simulink model "ModelMotS_dq_V2bis_FVC"  (R2018b)
settings: Solver=ode45  StartTime=0.0  StopTime=40  MaxStep=1e-4  RelTol=1e-4  EnableMultiTasking=on
values from neighbouring files (symbols this model uses):
  J = 0.045    [gen_sim_new_data_december.m]
  Lfr = 0.007    [gen_sim_new_data_december.m]
  Lfs = 0.007    [gen_sim_new_data_december.m]
  Lm = 0.153    [gen_sim_new_data_december.m]
  Lmt = 0.210    (= 0.21)    [gen_sim_new_data_december.m]
  Lr = 0.160    (= 0.16)    [gen_sim_new_data_december.m]
  Ls = 0.160    (= 0.16)    [gen_sim_new_data_december.m]
  np = 2    [gen_sim_new_data_december.m]
  P1 = 0.7    [gen_sim_new_data_december.m]
  P2 = 1.5    [gen_sim_new_data_december.m]
  Prinit = [ 0 ; 0 ]    [gen_sim_new_data_december.m]
  Psinit = [ 0 ; 0 ]    [gen_sim_new_data_december.m]
  Rr = 0.9    [gen_sim_new_data_december.m]
  Rs = 1.5    [gen_sim_new_data_december.m]
  thrinit = 0    [gen_sim_new_data_december.m]
  wL = 2*pi*0    (= 0)    [gen_sim_new_data_december.m]
  wrinit = 2*pi*0    (= 0)    [gen_sim_new_data_december.m]
undefined symbols (not defined in the file or in its folder): Data_Ts, DiscIntNeverNeededParam, Inom, Jm, Prdnom, SFC_Coeff, SLP_Coeff, Tpwm, Vnom, wCurr, wCurr_PI, wSpeed_PI, wSpeedEst, xiCurr_PI, xiSpeed_PI
libraries: simulink x5
(part 1 of 2)
settings Model: Creator=stbp106  LastModifiedBy=root
settings DataIOCC: LimitDataPoints=on  SaveFormat=Array
settings OptimizationCC: LifeSpan=inf
settings DebuggingCC: UnderspecifiedInitializationDetection=Classic  MergeDetectMultiDrivingBlocksExec=none  SolverPrmCheckMsg=warning  SFUnexpectedBacktrackingDiag=warning  SFNoUnconditionalDefaultTransitionDiag=warning  SFExecutionAtInitializationDiag=none
settings HardwareCC: ProdBitPerPointer=32  ProdBitPerSizeT=32  ProdBitPerPtrDiffT=32  ProdLargestAtomicFloat=None  ProdIntDivRoundTo=Undefined  ProdEndianess=Unspecified  ProdWordSize=32  ProdHWDeviceType=32-bit Generic
settings ModelReferenceCC: PropagateSignalLabelsOutOfModel=off
settings SFSimCC: SimUseLocalCustomCode=off
settings RTWCC: RTWUseLocalCustomCode=off
settings CodeAppCC: StateflowObjectComments=on
settings GRTTargetCC: TargetLangStandard=C89/C90 (ANSI)  GeneratePreprocessorConditionals=Disable all
settings ConfigComp: CovMetricSettings=dw  CovHtmlReporting=on  CovSaveCumulativeToWorkspaceVar=on  CovSaveSingleToWorkspaceVar=on  CovExternalEMLEnable=off  CovSFcnEnable=off

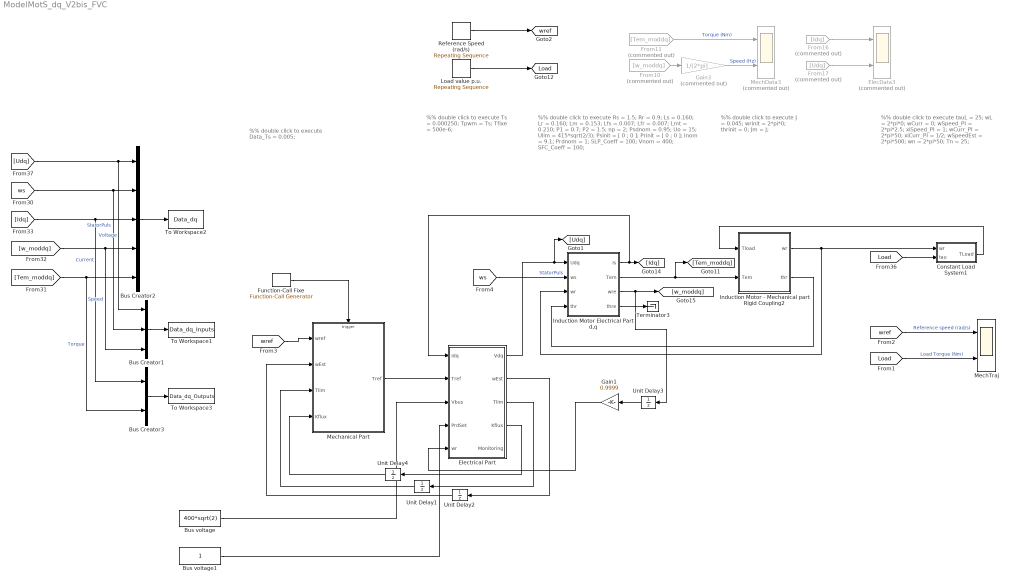
== system ModelMotS_dq_V2bis_FVC ==
  note: %% double click to execute
      |
      | Rs = 1.5; Rr = 0.9;
      | Ls = 0.160; Lr = 0.160; Lm = 0.153;
      | Lfs = 0.007; Lfr = 0.007; Lmt = 0.210; P1 = 0.7; P2 = 1.5;
      | np = 2;
      | Psdnom = 0.95; Uo = 15; Ulim = 415*sqrt(2/3);
      | Psinit = [ 0 ; 0 ]; Prinit = [ 0 ; 0 ];
      | Inom = 9.1; Prdnom = 1; SLP_Coeff = 100; Vnom = 400;
      | SFC_Coeff = 100;
  note: %% double click to execute
      |
      | J = 0.045;
      | wrinit = 2*pi*0;
      | thrinit = 0;
      | Jm = J;
  note: %% double click to execute
      |
      | tauL = 25;
      | wL = 2*pi*0;
      |
      | wCurr = 0;
      | wSpeed_PI = 2*pi*2.5; xiSpeed_PI = 1;
      | wCurr_PI = 2*pi*50; xiCurr_PI = 1/2;
      | wSpeedEst = 2*pi*500;
      |
      | wn = 2*pi*50;
      | Tn = 25;
  note: %% double click to execute
      |
      | Ts = 0.000250;
      | Tpwm = Ts;
      | Tfixe = 500e-6;
  note: %% double click to execute
      |
      | Data_Ts = 0.005;
  Bus Creator1 : BusCreator  Inputs=3
  Bus Creator2 : BusCreator  Inputs=5
  Bus Creator3 : BusCreator  Inputs=2
  Bus voltage : Constant  Value=400*sqrt(2)
  Bus voltage1 : Constant
  Constant Load System1 : Subsystem  Description=""
  ElecData3 : Scope  Commented=on  NumInputPorts=2
  Electrical Part : Subsystem
  From10 : From  Commented=on  GotoTag=w_moddq
  From11 : From  Commented=on  GotoTag=Tem_moddq
  From16 : From  Commented=on  GotoTag=Idq
  From17 : From  Commented=on  GotoTag=Udq
  Function-Call Fixe : simulink/Ports & Subsystems/Function-Call Generator  sample_time=Tfixe  numberOfIterations=1
  Gain1 : Gain  Gain=0.9999
  Gain3 : Gain  Commented=on  Gain=1/(2*pi)  SaturateOnIntegerOverflow=on  OutDataTypeStr=Inherit: Same as input  ParamDataTypeStr=Inherit: Same as input
  Induction Motor Electrical Part d,q : Subsystem  Description=""
  Induction Motor - Mechanical part Rigid Coupling2 : Subsystem  Description=""
  Load value p.u. : simulink/Sources/Repeating Sequence  rep_seq_t="[0        0.005         0.01        0.015         0.02        0.025         0.03        0.035         0.04        0.045         0.05        0.055         0.06        0.065         0.07        0.075         0.08        0.085         0.09        0.095          0.1        0.105         0.11        0.115         0.12        0.125         0.13        0.135         0.14        0.145         0.15        0.155         0.16        0.165         0.17        0.175         0.18        0.185         0.19        0.195          0.2        0.205         0.21        0.215         0.22        0.225         0.23        0.235         0.24        0.245         0.25        0.255         0.26        0.265         0.27        0.275         0.28        0.285         0.29        0.295          0.3        0.305         0.31        0.315         0.32        0.325         0.33        0.335         0.34        0.345         0.35        0.355         0.36        0.365         0.37        0.375         0.38        0.385         0.39        0.395          0.4        0.405         0.41        0.415         0.42        0.425         0.43        0.435         0.44        0.445         0.45        0.455         0.46        0.465         0.47        0.475         0.48        0.485         0.49        0.495          0.5        0.505         0.51        0.515         0.52        0.525         0.53        0.535         0.54        0.545         0.55        0.555         0.56        0.565         0.57        0.575         0.58        0.585         0.59        0.595          0.6        0.605         0.61        0.615         0.62        0.625         0.63        0.635         0.64        0.645         0.65        0.655         0.66        0.665         0.67        0.675         0.68        0.685         0.69        0.695          0.7        0.705         0.71        0.715         0.72        0.725         0.73        0.735         0.74        0.745         0.75        0.755         0.76        0.765         0.77        0.775         0.78        0.785         0.79        0.795          0.8        0.805         0.81        0.815         0.82        0.825         0.83        0.835         0.84        0.845         0.85        0.855         0.86        0.865         0.87        0.875         0.88        0.885         0.89        0.895          0.9        0.905         0.91        0.915         0.92        0.925         0.93        0.935         0.94        0.945         0.95        0.955         0.96        0.965         0.97        0.975         0.98        0.985         0.99        0.995            1        1.005         1.01        1.015         1.02        1.025         1.03        1.035         1.04        1.045         1.05        1.055         1.06        1.065         1.07        1.075         1.08        1.085         1.09        1.095          1.1        1.105         1.11        1.115         1.12        1.125         1.13        1.135         1.14        1.145         1.15        1.155         1.16        1.165         1.17        1.175         1.18        1.185         1.19        1.195          1.2        1.205         1.21        1.215         1.22        1.225         1.23        1.235         1.24        1.245         1.25        1.255         1.26        1.265         1.27        1.275         1.28        1.285         1.29        1.295          1.3        1.305         1.31        1.315         1.32        1.325         1.33        1.335         1.34        1.345         1.35        1.355         1.36        1.365         1.37        1.375         1.38        1.385         1.39        1.395          1.4        1.405         1.41        1.415         1.42        1.425         1.43        1.435         1.44        1.445         1.45        1.455         1.46        1.465         1.47        1.475         1.48        1.485         1.49        1.495          1.5        1.505         1.51        1.515         1.52        1.525         1.53        1.535 ...(+99990 chars)]"  rep_seq_y="[0            0            0            0            0            0            0            0            0            0            0            0            0            0            0            0            0            0            0            0            0            0            0            0            0            0            0            0            0            0            0            0            0            0            0            0            0            0            0            0            0            0            0            0            0            0            0            0            0            0            0            0            0            0            0            0            0            0            0            0            0            0            0            0            0            0            0            0            0            0            0            0            0            0            0            0            0            0            0            0            0            0            0            0            0            0            0            0            0            0            0            0            0            0            0            0            0            0            0            0            0            0            0            0            0            0            0            0            0            0            0            0            0            0            0            0            0            0            0            0            0            0            0            0            0            0            0            0            0            0            0            0            0            0            0            0            0            0            0            0            0            0            0            0            0            0            0            0            0            0            0            0            0            0            0            0            0            0            0            0            0            0            0            0            0            0            0            0            0            0            0            0            0            0            0            0            0            0            0            0            0            0            0            0            0            0            0            0            0            0            0            0            0            0            0            0            0            0            0            0            0            0            0            0            0            0            0            0            0            0            0            0            0            0            0            0            0            0            0            0            0            0            0            0            0            0            0            0            0            0            0            0            0            0            0            0            0            0            0            0            0            0            0            0            0            0            0            0            0            0            0            0            0            0            0            0            0            0            0            0            0            0            0            0            0            0            0            0            0            0            0            0            0            0            0            0            0            0            0            0            0            0            0            0            0            0            0            0            0            0            0            0            0            0            0            0            0            0            0            0            0            0            0            0            0            0            0            0 ...(+99990 chars)]"
  MechData3 : Scope  Commented=on  NumInputPorts=2
  MechTraj : Scope  NumInputPorts=2
  Mechanical Part : Subsystem
  Reference Speed (rad/s) : simulink/Sources/Repeating Sequence  rep_seq_t="[0        0.005         0.01        0.015         0.02        0.025         0.03        0.035         0.04        0.045         0.05        0.055         0.06        0.065         0.07        0.075         0.08        0.085         0.09        0.095          0.1        0.105         0.11        0.115         0.12        0.125         0.13        0.135         0.14        0.145         0.15        0.155         0.16        0.165         0.17        0.175         0.18        0.185         0.19        0.195          0.2        0.205         0.21        0.215         0.22        0.225         0.23        0.235         0.24        0.245         0.25        0.255         0.26        0.265         0.27        0.275         0.28        0.285         0.29        0.295          0.3        0.305         0.31        0.315         0.32        0.325         0.33        0.335         0.34        0.345         0.35        0.355         0.36        0.365         0.37        0.375         0.38        0.385         0.39        0.395          0.4        0.405         0.41        0.415         0.42        0.425         0.43        0.435         0.44        0.445         0.45        0.455         0.46        0.465         0.47        0.475         0.48        0.485         0.49        0.495          0.5        0.505         0.51        0.515         0.52        0.525         0.53        0.535         0.54        0.545         0.55        0.555         0.56        0.565         0.57        0.575         0.58        0.585         0.59        0.595          0.6        0.605         0.61        0.615         0.62        0.625         0.63        0.635         0.64        0.645         0.65        0.655         0.66        0.665         0.67        0.675         0.68        0.685         0.69        0.695          0.7        0.705         0.71        0.715         0.72        0.725         0.73        0.735         0.74        0.745         0.75        0.755         0.76        0.765         0.77        0.775         0.78        0.785         0.79        0.795          0.8        0.805         0.81        0.815         0.82        0.825         0.83        0.835         0.84        0.845         0.85        0.855         0.86        0.865         0.87        0.875         0.88        0.885         0.89        0.895          0.9        0.905         0.91        0.915         0.92        0.925         0.93        0.935         0.94        0.945         0.95        0.955         0.96        0.965         0.97        0.975         0.98        0.985         0.99        0.995            1        1.005         1.01        1.015         1.02        1.025         1.03        1.035         1.04        1.045         1.05        1.055         1.06        1.065         1.07        1.075         1.08        1.085         1.09        1.095          1.1        1.105         1.11        1.115         1.12        1.125         1.13        1.135         1.14        1.145         1.15        1.155         1.16        1.165         1.17        1.175         1.18        1.185         1.19        1.195          1.2        1.205         1.21        1.215         1.22        1.225         1.23        1.235         1.24        1.245         1.25        1.255         1.26        1.265         1.27        1.275         1.28        1.285         1.29        1.295          1.3        1.305         1.31        1.315         1.32        1.325         1.33        1.335         1.34        1.345         1.35        1.355         1.36        1.365         1.37        1.375         1.38        1.385         1.39        1.395          1.4        1.405         1.41        1.415         1.42        1.425         1.43        1.435         1.44        1.445         1.45        1.455         1.46        1.465         1.47        1.475         1.48        1.485         1.49        1.495          1.5        1.505         1.51        1.515         1.52        1.525         1.53        1.535 ...(+99990 chars)]"  rep_seq_y="[62.8319      62.8319      62.8319      62.8319      62.8319      62.8319      62.8319      62.8319      62.8319      62.8319      62.8319      62.8319      62.8319      62.8319      62.8319      62.8319      62.8319      62.8319      62.8319      62.8319      62.8319      62.8319      62.8319      62.8319      62.8319      62.8319      62.8319      62.8319      62.8319      62.8319      62.8319      62.8319      62.8319      62.8319      62.8319      62.8319      62.8319      62.8319      62.8319      62.8319      62.8319      62.8319      62.8319      62.8319      62.8319      62.8319      62.8319      62.8319      62.8319      62.8319      62.8319      62.8319      62.8319      62.8319      62.8319      62.8319      62.8319      62.8319      62.8319      62.8319      62.8319      62.8319      62.8319      62.8319      62.8319      62.8319      62.8319      62.8319      62.8319      62.8319      62.8319      62.8319      62.8319      62.8319      62.8319      62.8319      62.8319      62.8319      62.8319      62.8319      62.8319      62.8319      62.8319      62.8319      62.8319      62.8319      62.8319      62.8319      62.8319      62.8319      62.8319      62.8319      62.8319      62.8319      62.8319      62.8319      62.8319      62.8319      62.8319      62.8319      62.8319      62.8319      62.8319      62.8319      62.8319      62.8319      62.8319      62.8319      62.8319      62.8319      62.8319      62.8319      62.8319      62.8319      62.8319      62.8319      62.8319      62.8319      62.8319      62.8319      62.8319      62.8319      62.8319      62.8319      62.8319      62.8319      62.8319      62.8319      62.8319      62.8319      62.8319      62.8319      62.8319      62.8319      62.8319      62.8319      62.8319      62.8319      62.8319      62.8319      62.8319      62.8319      62.8319      62.8319      62.8319      62.8319      62.8319      62.8319      62.8319      62.8319      62.8319      62.8319      62.8319      62.8319      62.8319      62.8319      62.8319      62.8319      62.8319      62.8319      62.8319      62.8319      62.8319      62.8319      62.8319      62.8319      62.8319      62.8319      62.8319      62.8319      62.8319      62.8319      62.8319      62.8319      62.8319      62.8319      62.8319      62.8319      62.8319      62.8319      62.8319      62.8319      62.8319      62.8319      62.8319      62.8319      62.8319      62.8319      62.8319      62.8319      62.8319      62.8319      62.8319      62.8319      62.8319      62.8319      62.8319      62.8319      62.8319      62.8319      62.8319      62.8319      62.8319      62.8319      62.8319      62.8319      62.8319      62.8319      62.8319      62.8319      62.8319      62.8319      62.8319      62.8319      62.8319      62.8319      62.8319      62.8319      62.8319      62.8319      62.8319      62.8319      62.8319      62.8319      62.8319      62.8319      62.8319      62.8319      62.8319      62.8319      62.8319      62.8319      62.8319      62.8319      62.8319      62.8319      62.8319      62.8319      62.8319      62.8319      62.8319      62.8319      62.8319      62.8319      62.8319      62.8319      62.8319      62.8319      62.8319      62.8319      62.8319      62.8319      62.8319      62.8319      62.8319      62.8319      62.8319      62.8319      62.8319      62.8319      62.8319      62.8319      62.8319      62.8319      62.8319      62.8319      62.8319      62.8319      62.8319      62.8319      62.8319      62.8319      62.8319      62.8319      62.8319      62.8319      62.8319      62.8319      62.8319      62.8319      62.8319      62.8319      62.8319      62.8319      62.8319      62.8319      62.8319      62.8319      62.8319      62.8319      62.8319      62.8319      62.8319      62.8319      62.8319      62.8319      62.8319      62.8319      62.8319      62.8319      62.8319      62.8319      62.8319      62.8319      62.8319      62.8319      62.8319      62.8319 ...(+99996 chars)]"
  Terminator3 : Terminator
  To Workspace1 : ToWorkspace  VariableName=Data_dq_Inputs  SaveFormat=Timeseries  SampleTime=Data_Ts
  To Workspace2 : ToWorkspace  VariableName=Data_dq  SaveFormat=Timeseries  SampleTime=Data_Ts
  To Workspace3 : ToWorkspace  VariableName=Data_dq_Outputs  SaveFormat=Timeseries  SampleTime=Data_Ts
  Unit Delay{1..4} (4 alike) : UnitDelay  SampleTime=-1
  tag scope: Load=global, wref=global
  wires:
  Reference Speed (rad/s)/1 -> [wref]
  Induction Motor - Mechanical part Rigid Coupling2/2(thr) -> Induction Motor Electrical Part d,q/4(thr)
  Induction Motor Electrical Part d,q/2(Tem) -> [Tem_moddq], Induction Motor - Mechanical part Rigid Coupling2/2(Tem)
  Induction Motor - Mechanical part Rigid Coupling2/1(wr) -> Constant Load System1/1(wr), Induction Motor Electrical Part d,q/3(wr)
  Induction Motor Electrical Part d,q/4(thre) -> Terminator3/1
  Constant Load System1/1(TLoad) -> Induction Motor - Mechanical part Rigid Coupling2/1(Tload)
  Induction Motor Electrical Part d,q/1(Is) -> Electrical Part/1(Idq), [Idq]
  Induction Motor Electrical Part d,q/3(wre) -> Unit Delay3/1, [w_moddq]
  [Load] -> Constant Load System1/2(tau)
  From16/1 -> ElecData3/1
  From17/1 -> ElecData3/2
  From10/1 -> Gain3/1
  From11/1 -> MechData3/1  "Torque (Nm)"
  Gain3/1 -> MechData3/2  "Speed (Hz)"
  Load value p.u./1 -> [Load]
  [Udq] -> Bus Creator1/1, Bus Creator2/1  "Voltage"
  [Idq] -> Bus Creator3/1, Bus Creator2/3  "Current"
  [w_moddq] -> Bus Creator1/3, Bus Creator2/4  "Speed"
  [Tem_moddq] -> Bus Creator3/2, Bus Creator2/5  "Torque"
  Bus Creator2/1 -> To Workspace2/1
  [ws] -> Bus Creator1/2, Bus Creator2/2  "StatorPuls"
  [Load] -> MechTraj/2  "Load Torque (Nm)"
  [wref] -> MechTraj/1  "Reference speed (rad/s)"
  Mechanical Part/1(Tref) -> Electrical Part/2(Tref)
  [wref] -> Mechanical Part/1(wref)
  Electrical Part/2(wEst) -> Unit Delay2/1
  Electrical Part/3(Tlim) -> Unit Delay1/1
  Electrical Part/4(Kflux) -> Unit Delay4/1
  Unit Delay4/1 -> Mechanical Part/4(Kflux)
  Unit Delay1/1 -> Mechanical Part/3(Tlim)
  Unit Delay2/1 -> Mechanical Part/2(wEst)
  Electrical Part/1(Vdq) -> [Udq], Induction Motor Electrical Part d,q/1(Udq)
  [ws] -> Induction Motor Electrical Part d,q/2(ws)  "StatorPuls"
  Unit Delay3/1 -> Gain1/1
  Gain1/1 -> Electrical Part/5(wr)
  Bus voltage/1 -> Electrical Part/3(Vbus)
  Bus voltage1/1 -> Electrical Part/4(PrdSet)
  Function-Call Fixe/1 -> Mechanical Part/Trigger
  Bus Creator3/1 -> To Workspace3/1
  Bus Creator1/1 -> To Workspace1/1
